simulink model "s9_10"  (Simulink 6.6)
settings: Solver=ode23  SolverMode=SingleTasking  StartTime=0.0  StopTime=t_d  MaxStep=Tc  RelTol=1e-8  AbsTol=1e-8
values from neighbouring files (symbols this model uses):
  Cp = [0 0;0 1/4e3]    [i9_10.m]
  F_v = K_r*diag([0.01 0.01])*K_r    [i9_10.m]
  g = 9.81    [i9_10.m]
  G_f = inv (S_f'*Ch*S_f)*S_f'    [i9_10.m]
  h_d = [0;- 50]    [i9_10.m]
  K_Dl = 16    [i9_10.m]
  K_Inu = 100    [i9_10.m]
  K_Pl = 100    [i9_10.m]
  K_Pnu = 16    [i9_10.m]
  o_r = [1;0]    [i9_10.m]
  pi_l = pi_m    [i9_10.m]
  pS_f = inv(S_f'*Ch*S_f)*S_f'*Ch    [i9_10.m]
  pS_v = inv(S_v'*Kh*S_v)*S_v'*Kh    [i9_10.m]
  q_i = inv_k2u(a,p_0)    [i9_10.m]
  R_c = [cos(pi/4)  -sin(pi/4) ... (first row only)    [i9_10.m]
  S_f = [0;1]    [i9_10.m]
  S_v = [1;0]    [i9_10.m]
  Tc = 0.001    [i9_10.m]
  Ts = Tc    (= 0.001)    [i9_10.m]
undefined symbols (not defined in the file or in its folder): a, DiscIntNeverNeededParam, iner, iner_l, pi_m
settings Model: Creator=luigivillani  LastModifiedBy=luigivillani  ExtModeAutoUpdateStatusClock=off
settings DataIOCC: LimitDataPoints=off  SaveOutput=off  SaveTime=off
settings OptimizationCC: BlockReduction=off  BooleanDataType=off
settings DebuggingCC: SignalResolutionControl=TryResolveAllWithWarning  SolverPrmCheckMsg=none  MultiTaskDSMMsg=warning  MultiTaskCondExecSysMsg=none  StrictBusMsg=None
settings HardwareCC: TargetUnknown=on
settings RTWCC: IncludeERTFirstTime=on

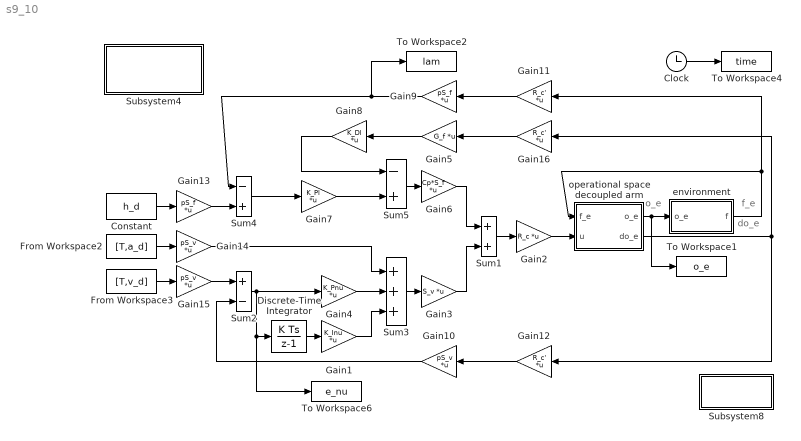
== system s9_10 ==
  note: do_e
  note: f_e
  note: o_e
  Clock : Clock
      settings: Decimation=10
  Constant : Constant  Value=h_d
  Discrete-Time Integrator : DiscreteIntegrator  SampleTime=Tc  ICPrevOutput=DiscIntNeverNeededParam  ICPrevScaledInput=DiscIntNeverNeededParam
  From Workspace2 : FromWorkspace  VariableName=[T,a_d]  SampleTime=Tc
  From Workspace3 : FromWorkspace  VariableName=[T,v_d]  SampleTime=Tc
  Gain1 : Gain  Gain=K_Inu  Multiplication=Matrix(K*u)  SampleTime=Tc
      mask Display: disp('K_Inu')
  Gain10 : Gain  Orientation=left  Gain=pS_v  Multiplication=Matrix(K*u)  SampleTime=Tc
      mask Display: disp('pS_v')
  Gain11 : Gain  Orientation=left  Gain=R_c'  Multiplication=Matrix(K*u)  SampleTime=Tc
      mask Display: disp('trR_c')
  Gain12 : Gain  Orientation=left  Gain=R_c'  Multiplication=Matrix(K*u)  SampleTime=Tc
      mask Display: disp('trR_c')
  Gain13 : Gain  Gain=pS_f  Multiplication=Matrix(K*u)  SampleTime=Tc
      mask Display: disp('pS_f')
  Gain14 : Gain  Gain=pS_v  Multiplication=Matrix(K*u)  SampleTime=Tc
      mask Display: disp('pS_v')
  Gain15 : Gain  Gain=pS_v  Multiplication=Matrix(K*u)  SampleTime=Tc
      mask Display: disp('pS_v')
  Gain16 : Gain  Orientation=left  Gain=R_c'  Multiplication=Matrix(K*u)  SampleTime=Tc
      mask Display: disp('trR_c')
  Gain2 : Gain  Gain=R_c  Multiplication=Matrix(K*u)  SampleTime=Tc
      mask Display: disp('R_c')
  Gain3 : Gain  Gain=S_v  Multiplication=Matrix(K*u)  SampleTime=Tc
      mask Display: disp('S_v')
  Gain4 : Gain  Gain=K_Pnu  Multiplication=Matrix(K*u)  SampleTime=Tc
      mask Display: disp('K_Pnu')
  Gain5 : Gain  Orientation=left  Gain=G_f  Multiplication=Matrix(K*u)  SampleTime=Tc
      mask Display: disp('G_f')
  Gain6 : Gain  Gain=Cp*S_f  Multiplication=Matrix(K*u)  SampleTime=Tc
      mask Display: disp('C''S_f')
  Gain7 : Gain  Gain=K_Pl  Multiplication=Matrix(K*u)  SampleTime=Tc
      mask Display: disp('K_Pl')
  Gain8 : Gain  Orientation=left  Gain=K_Dl  Multiplication=Matrix(K*u)  SampleTime=Tc
      mask Display: disp('K_Dl')
  Gain9 : Gain  Orientation=left  Gain=pS_f  Multiplication=Matrix(K*u)  SampleTime=Tc
      mask Display: disp('pS_f')
  Subsystem4 : Subsystem
      settings: OpenFcn=clear all;i9_10;
      mask Display: disp('variables\ninitialization')
  Subsystem8 : Subsystem  Orientation=left
      settings: OpenFcn=p9_10;
      mask Display: disp('plot')
  Sum1 : Sum  SaturateOnIntegerOverflow=on  InputSameDT=on
  Sum2 : Sum  Inputs=+-  SaturateOnIntegerOverflow=on  InputSameDT=on
  Sum3 : Sum  Inputs=+++  SaturateOnIntegerOverflow=on  InputSameDT=on
  Sum4 : Sum  Inputs=-+  SaturateOnIntegerOverflow=on  InputSameDT=on
  Sum5 : Sum  Inputs=-+  SaturateOnIntegerOverflow=on  InputSameDT=on
  To Workspace1 : ToWorkspace  VariableName=o_e  SampleTime=Ts  SaveFormat=Array
      settings: MaxDataPoints=5001
  To Workspace2 : ToWorkspace  VariableName=lam  SampleTime=Ts  SaveFormat=Array
      settings: MaxDataPoints=5001
  To Workspace4 : ToWorkspace  VariableName=time  SampleTime=Ts  SaveFormat=Array
      settings: MaxDataPoints=5001
  To Workspace6 : ToWorkspace  VariableName=e_nu  SampleTime=Ts  SaveFormat=Array
      settings: MaxDataPoints=5001
  environment : Subsystem
      mask Display: disp('K''(o_e-o_r)')
  operational space decoupled arm : Subsystem
      mask Display: disp('u = ddo_e')
  wires:
  Sum2/1 -> To Workspace6/1, Discrete-Time Integrator/1, Gain4/1
  environment/1(f) -> Gain11/1, operational space decoupled arm/1(f_e)
  Clock/1 -> To Workspace4/1
  operational space decoupled arm/1(o_e) -> environment/1(o_e), To Workspace1/1
  operational space decoupled arm/2(do_e) -> Gain12/1, Gain16/1
  Gain4/1 -> Sum3/2
  Gain2/1 -> operational space decoupled arm/2(u)
  Gain1/1 -> Sum3/3
  Discrete-Time Integrator/1 -> Gain1/1
  Sum3/1 -> Gain3/1
  Gain3/1 -> Sum1/2
  Sum4/1 -> Gain7/1
  Gain7/1 -> Sum5/2
  Sum5/1 -> Gain6/1
  Gain6/1 -> Sum1/1
  Sum1/1 -> Gain2/1
  Gain9/1 -> Sum4/1, To Workspace2/1
  Gain10/1 -> Sum2/2
  Gain5/1 -> Gain8/1
  Gain8/1 -> Sum5/1
  Gain11/1 -> Gain9/1
  Gain12/1 -> Gain10/1
  Constant/1 -> Gain13/1
  Gain13/1 -> Sum4/2
  From Workspace2/1 -> Gain14/1
  Gain14/1 -> Sum3/1
  From Workspace3/1 -> Gain15/1
  Gain15/1 -> Sum2/1
  Gain16/1 -> Gain5/1

== system s9_10/Subsystem4 ==
  note: start

== system s9_10/Subsystem8 ==
  note: start

== system s9_10/environment ==
  o_e : Inport
  Matrix gain. : StateSpace  A=[]  B=[]  C=[]  D=K  mask(Matrix gain){@1=K}
      mask prompts: @1 "Gain matrix:"
      mask help: Matrix Gain.
      mask init:
      | K = @1;
      mask Help: Multiplies input vector by entered matrix to produce output vector (y=Au).
      mask Display: disp('K')
  Sum1 : Sum  Inputs=+-  SaturateOnIntegerOverflow=on  InputSameDT=on
  xo : Constant  Value=o_r
  f : Outport  InitialOutput=0
  wires:
  xo/1 -> Sum1/2
  Sum1/1 -> Matrix gain./1
  Matrix gain./1 -> f/1
  o_e/1 -> Sum1/1

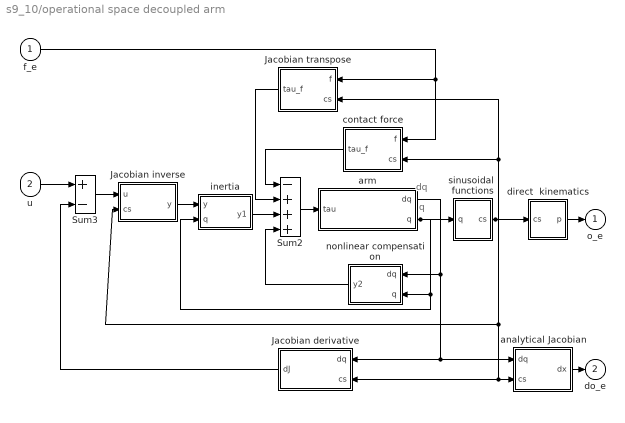
== system s9_10/operational space decoupled arm ==
  note: q
  note: dq
  f_e : Inport
  u : Inport  Port=2
  Jacobian derivative : Subsystem  Orientation=left
      mask Display: disp('dJ_a(q,dq)')
  Jacobian inverse : Subsystem
      mask Display: disp('inv(J_a(q))')
  Jacobian transpose : Subsystem  Orientation=left
      mask Display: disp('tr(J_a(q))')
  Sum2 : Sum  Inputs=-+++  SaturateOnIntegerOverflow=on  InputSameDT=on
  Sum3 : Sum  Inputs=+-  SaturateOnIntegerOverflow=on  InputSameDT=on
  analytical Jacobian : Subsystem
      mask Display: disp('J_a(q)')
  arm : Subsystem
      mask Display: disp('inv(B(q))(tau-tau'')')
  contact force : Subsystem  Orientation=left
      mask Display: disp('tr(J_a(q))f')
  direct  kinematics : Subsystem
      mask Display: disp('k(q)')
  inertia : Subsystem
      mask Display: disp('B(q)')
  nonlinear compensation : Subsystem  Orientation=left
      mask Display: disp('n(q,dq)')
  sinusoidal  functions : Subsystem
      mask Display: disp('cs(q)')
  o_e : Outport  InitialOutput=0
  do_e : Outport  Port=2  InitialOutput=0
  wires:
  Jacobian inverse/1(y) -> inertia/1(y)
  Sum2/1 -> arm/1(tau)
  arm/1(dq) -> analytical Jacobian/1(dq), Jacobian derivative/1(dq), nonlinear compensation/1(dq)
  direct  kinematics/1(p) -> o_e/1
  analytical Jacobian/1(dx) -> do_e/1
  Sum3/1 -> Jacobian inverse/1(u)
  arm/2("q ") -> sinusoidal  functions/1(q), nonlinear compensation/2(q), inertia/2(q)
  contact force/1(tau_f) -> Sum2/1
  sinusoidal  functions/1(cs) -> direct  kinematics/1(cs), contact force/2(cs), Jacobian transpose/2(cs), analytical Jacobian/2(cs), Jacobian derivative/2(cs), Jacobian inverse/2(cs)
  u/1 -> Sum3/1
  Jacobian derivative/1(dJ) -> Sum3/2
  nonlinear compensation/1(y2) -> Sum2/4
  inertia/1(y1) -> Sum2/3
  Jacobian transpose/1(tau_f) -> Sum2/2
  f_e/1 -> Jacobian transpose/1(f), contact force/1(f)

== system s9_10/operational space decoupled arm/Jacobian derivative ==
  dq : Inport
  cs : Inport  Port=2
  MATLAB Fcn : MATLABFcn  MATLABFcn=dJ_a  OutputDimensions=2  SampleTime=Tc
      mask Display: disp('dJ_a(q,dq)dq')
  Mux : Mux  Inputs=[2,4]
  dJ : Outport  InitialOutput=0
  wires:
  dq/1 -> Mux/1
  cs/1 -> Mux/2
  Mux/1 -> MATLAB Fcn/1
  MATLAB Fcn/1 -> dJ/1

== system s9_10/operational space decoupled arm/Jacobian inverse ==
  u : Inport
  cs : Inport  Port=2
  MATLAB Fcn : MATLABFcn  MATLABFcn=invJ_a  OutputDimensions=2  SampleTime=Tc
      mask Display: disp('inv(J_a(q))')
  Mux : Mux  Inputs=[2,4]
  y : Outport  InitialOutput=0
  wires:
  MATLAB Fcn/1 -> y/1
  Mux/1 -> MATLAB Fcn/1
  cs/1 -> Mux/2
  u/1 -> Mux/1

== system s9_10/operational space decoupled arm/Jacobian transpose ==
  f : Inport
  cs : Inport  Port=2
  MATLAB Fcn : MATLABFcn  MATLABFcn=trJ_a  OutputDimensions=2  SampleTime=Tc
      mask Display: disp('J''_a(q)f')
  Mux : Mux  Inputs=[2,4]
  tau_f : Outport  InitialOutput=0
  wires:
  MATLAB Fcn/1 -> tau_f/1
  Mux/1 -> MATLAB Fcn/1
  f/1 -> Mux/1
  cs/1 -> Mux/2

== system s9_10/operational space decoupled arm/analytical Jacobian ==
  dq : Inport
  cs : Inport  Port=2
  MATLAB Fcn : MATLABFcn  MATLABFcn=J_adq  OutputDimensions=2
      mask Display: disp('J_a(q)dq')
  Mux : Mux  Inputs=[2,4]
  dx : Outport  InitialOutput=0
  wires:
  dq/1 -> Mux/1
  Mux/1 -> MATLAB Fcn/1
  MATLAB Fcn/1 -> dx/1
  cs/1 -> Mux/2

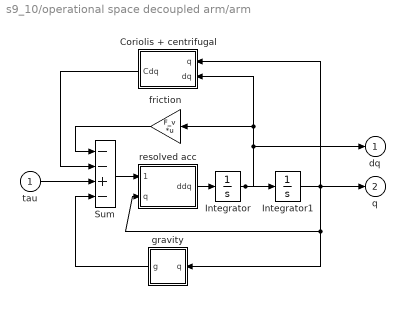
== system s9_10/operational space decoupled arm/arm ==
  tau : Inport
  Coriolis + centrifugal : Subsystem  Orientation=left
      mask Display: disp('C(q,dq)dq')
  Integrator : Integrator  InitialCondition=[0 0]  ZeroCross=off
  Integrator1 : Integrator  InitialCondition=q_i  ZeroCross=off
  Sum : Sum  Inputs=--+-  SaturateOnIntegerOverflow=on  InputSameDT=on
  friction : Gain  Orientation=left  Gain=F_v  Multiplication=Matrix(K*u)  SaturateOnIntegerOverflow=on
      mask Display: disp('F_v')
  gravity : Subsystem  Orientation=left
      mask Display: disp('g(q)')
  resolved acc : Subsystem
      mask Display: disp('inv(B(q))')
  dq : Outport  InitialOutput=0
  "q " : Outport  Port=2  InitialOutput=0
  wires:
  Coriolis + centrifugal/1(Cdq) -> Sum/2
  tau/1 -> Sum/3
  Integrator1/1 -> Coriolis + centrifugal/1(q), resolved acc/2(q), gravity/1(q), "q "/1
  resolved acc/1(ddq) -> Integrator/1
  Integrator/1 -> Integrator1/1, dq/1, Coriolis + centrifugal/2(dq), friction/1
  Sum/1 -> resolved acc/1(tau-tau')
  friction/1 -> Sum/1
  gravity/1(g) -> Sum/4

== system s9_10/operational space decoupled arm/contact force ==
  f : Inport
  cs : Inport  Port=2
  MATLAB Fcn : MATLABFcn  MATLABFcn=trJ_a  OutputDimensions=2
      mask Display: disp('J''_a(q)f')
  Mux : Mux  Inputs=[2,4]
  tau_f : Outport  InitialOutput=0
  wires:
  f/1 -> Mux/1
  cs/1 -> Mux/2
  Mux/1 -> MATLAB Fcn/1
  MATLAB Fcn/1 -> tau_f/1

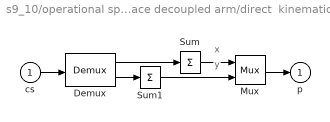
== system s9_10/operational space decoupled arm/direct  kinematics ==
  note: x
  note: y
  cs : Inport
  Demux : Demux  Outputs=[2,2]
  Mux : Mux  Inputs=2
  Sum : Sum  Inputs=+  SaturateOnIntegerOverflow=on  InputSameDT=on
  Sum1 : Sum  Inputs=+  SaturateOnIntegerOverflow=on  InputSameDT=on
  p : Outport  InitialOutput=0
  wires:
  Sum1/1 -> Mux/2
  Sum/1 -> Mux/1
  Demux/2 -> Sum1/1
  Demux/1 -> Sum/1
  cs/1 -> Demux/1
  Mux/1 -> p/1

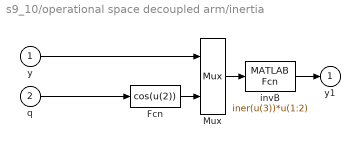
== system s9_10/operational space decoupled arm/inertia ==
  y : Inport
  q : Inport  Port=2
  Fcn : Fcn  Expr=cos(u(2))  SampleTime=Tc
  Mux : Mux  Inputs=[2,1]
  "invB " : MATLABFcn  MATLABFcn=iner(u(3))*u(1:2)  OutputDimensions=2  SampleTime=Tc
      mask Display: disp('B(q)y')
  y1 : Outport  InitialOutput=0
  wires:
  Fcn/1 -> Mux/2
  "invB "/1 -> y1/1
  Mux/1 -> "invB "/1
  q/1 -> Fcn/1
  y/1 -> Mux/1

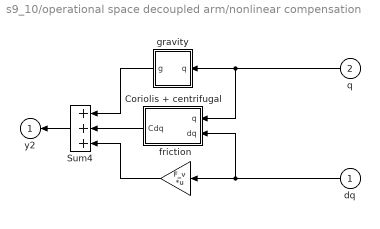
== system s9_10/operational space decoupled arm/nonlinear compensation ==
  dq : Inport  Orientation=left
  q : Inport  Orientation=left  Port=2
  Coriolis + centrifugal : Subsystem  Orientation=left
      mask Display: disp('C(q,dq)dq')
  Sum4 : Sum  Orientation=left  Inputs=+++  SaturateOnIntegerOverflow=on  InputSameDT=on
  friction : Gain  Orientation=left  Gain=F_v  Multiplication=Matrix(K*u)  SampleTime=Tc  SaturateOnIntegerOverflow=on
      mask Display: disp('F_v')
  gravity : Subsystem  Orientation=left
      mask Display: disp('g(q)')
  y2 : Outport  Orientation=left  InitialOutput=0
  wires:
  gravity/1(g) -> Sum4/1
  Sum4/1 -> y2/1
  friction/1 -> Sum4/3
  q/1 -> gravity/1(q), Coriolis + centrifugal/1(q)
  dq/1 -> Coriolis + centrifugal/2(dq), friction/1
  Coriolis + centrifugal/1(Cdq) -> Sum4/2

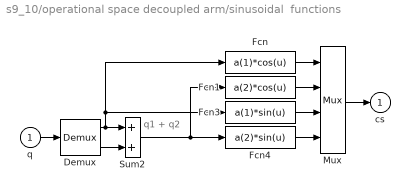
== system s9_10/operational space decoupled arm/sinusoidal  functions ==
  note: q1 + q2
  q : Inport
  Demux : Demux  Outputs=2
  Fcn : Fcn  Expr=a(1)*cos(u)
  Fcn1 : Fcn  Expr=a(2)*cos(u)
  Fcn3 : Fcn  Expr=a(1)*sin(u)
  Fcn4 : Fcn  Expr=a(2)*sin(u)
  Mux : Mux
  Sum2 : Sum  SaturateOnIntegerOverflow=on  InputSameDT=on
  cs : Outport  InitialOutput=0
  wires:
  q/1 -> Demux/1
  Fcn4/1 -> Mux/4
  Fcn3/1 -> Mux/3
  Fcn1/1 -> Mux/2
  Sum2/1 -> Fcn1/1, Fcn4/1
  Demux/2 -> Sum2/2
  Demux/1 -> Fcn/1, Fcn3/1, Sum2/1
  Mux/1 -> cs/1
  Fcn/1 -> Mux/1

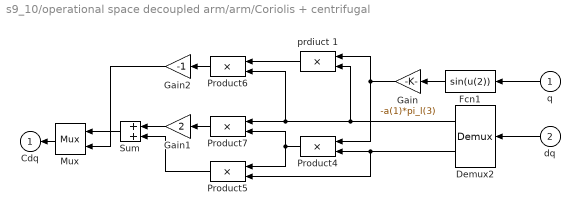
== system s9_10/operational space decoupled arm/arm/Coriolis + centrifugal ==
  q : Inport  Orientation=left
  dq : Inport  Orientation=left  Port=2
  Demux2 : Demux  Orientation=left  Outputs=2
  Fcn1 : Fcn  Orientation=left  Expr=sin(u(2))
  Gain : Gain  Orientation=left  Gain=-a(1)*pi_l(3)  SaturateOnIntegerOverflow=on
      mask Display: disp('k_3')
  Gain1 : Gain  Orientation=left  Gain=2  SaturateOnIntegerOverflow=on
  Gain2 : Gain  Orientation=left  Gain=-1  SaturateOnIntegerOverflow=on
  Mux : Mux  Orientation=left  Inputs=2
  Product{4..7} (4 alike) : Product  Orientation=left  SaturateOnIntegerOverflow=on  RndMeth=Zero  InputSameDT=on
  Sum : Sum  Orientation=left  SaturateOnIntegerOverflow=on  InputSameDT=on
  prdiuct 1 : Product  Orientation=left  SaturateOnIntegerOverflow=on  RndMeth=Zero  InputSameDT=on
  Cdq : Outport  Orientation=left  InitialOutput=0
  wires:
  dq/1 -> Demux2/1
  Gain2/1 -> Mux/2
  Product6/1 -> Gain2/1
  Mux/1 -> Cdq/1
  Sum/1 -> Mux/1
  Product5/1 -> Sum/2
  Gain1/1 -> Sum/1
  Product7/1 -> Gain1/1
  Demux2/1 -> prdiuct 1/2, Product6/2, Product7/1
  Demux2/2 -> Product4/2, Product5/2
  prdiuct 1/1 -> Product6/1
  Gain/1 -> prdiuct 1/1, Product4/1
  Fcn1/1 -> Gain/1
  q/1 -> Fcn1/1
  Product4/1 -> Product5/1, Product7/2

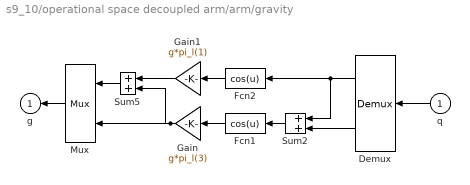
== system s9_10/operational space decoupled arm/arm/gravity ==
  q : Inport  Orientation=left
  Demux : Demux  Orientation=left  Outputs=2
  Fcn1 : Fcn  Orientation=left  Expr=cos(u)
  Fcn2 : Fcn  Orientation=left  Expr=cos(u)
  Gain : Gain  Orientation=left  Gain=g*pi_l(3)  SaturateOnIntegerOverflow=on
      mask Display: disp('k_2')
  Gain1 : Gain  Orientation=left  Gain=g*pi_l(1)  SaturateOnIntegerOverflow=on
      mask Display: disp('k_1')
  Mux : Mux  Orientation=left  Inputs=2
  Sum2 : Sum  Orientation=left  SaturateOnIntegerOverflow=on  InputSameDT=on
  Sum5 : Sum  Orientation=left  SaturateOnIntegerOverflow=on  InputSameDT=on
  g : Outport  Orientation=left  InitialOutput=0
  wires:
  q/1 -> Demux/1
  Demux/2 -> Sum2/2
  Sum2/1 -> Fcn1/1
  Fcn1/1 -> Gain/1
  Fcn2/1 -> Gain1/1
  Demux/1 -> Fcn2/1, Sum2/1
  Gain1/1 -> Sum5/1
  Sum5/1 -> Mux/1
  Gain/1 -> Sum5/2, Mux/2
  Mux/1 -> g/1

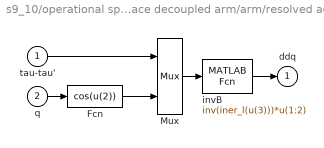
== system s9_10/operational space decoupled arm/arm/resolved acc ==
  tau-tau' : Inport
  q : Inport  Port=2
  Fcn : Fcn  Expr=cos(u(2))
  Mux : Mux  Inputs=[2,1]
  "invB " : MATLABFcn  MATLABFcn=inv(iner_l(u(3)))*u(1:2)  OutputDimensions=2
      mask Display: disp('inv(B(q))')
  ddq : Outport  InitialOutput=0
  wires:
  Fcn/1 -> Mux/2
  q/1 -> Fcn/1
  "invB "/1 -> ddq/1
  tau-tau'/1 -> Mux/1
  Mux/1 -> "invB "/1

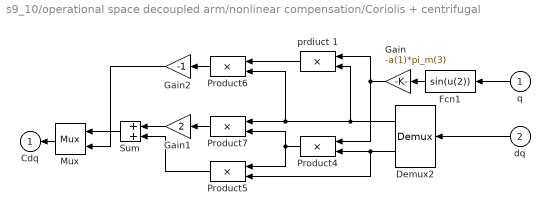
== system s9_10/operational space decoupled arm/nonlinear compensation/Coriolis + centrifugal ==
  q : Inport  Orientation=left
  dq : Inport  Orientation=left  Port=2
  Demux2 : Demux  Orientation=left  Outputs=2
  Fcn1 : Fcn  Orientation=left  Expr=sin(u(2))  SampleTime=Tc
  Gain : Gain  Orientation=left  Gain=-a(1)*pi_m(3)  SaturateOnIntegerOverflow=on
      mask Display: disp('k_3')
  Gain1 : Gain  Orientation=left  Gain=2  SaturateOnIntegerOverflow=on
  Gain2 : Gain  Orientation=left  Gain=-1  SaturateOnIntegerOverflow=on
  Mux : Mux  Orientation=left  Inputs=2
  Product{4..7} (4 alike) : Product  Orientation=left  SampleTime=Tc  SaturateOnIntegerOverflow=on  RndMeth=Zero  InputSameDT=on
  Sum : Sum  Orientation=left  SaturateOnIntegerOverflow=on  InputSameDT=on
  prdiuct 1 : Product  Orientation=left  SampleTime=Tc  SaturateOnIntegerOverflow=on  RndMeth=Zero  InputSameDT=on
  Cdq : Outport  Orientation=left  InitialOutput=0
  wires:
  Product4/1 -> Product5/1, Product7/2
  Demux2/1 -> prdiuct 1/2, Product6/2, Product7/1
  Fcn1/1 -> Gain/1
  Gain/1 -> prdiuct 1/1, Product4/1
  prdiuct 1/1 -> Product6/1
  Product7/1 -> Gain1/1
  Gain1/1 -> Sum/1
  Product5/1 -> Sum/2
  Sum/1 -> Mux/1
  Mux/1 -> Cdq/1
  Product6/1 -> Gain2/1
  Gain2/1 -> Mux/2
  q/1 -> Fcn1/1
  dq/1 -> Demux2/1
  Demux2/2 -> Product4/2, Product5/2

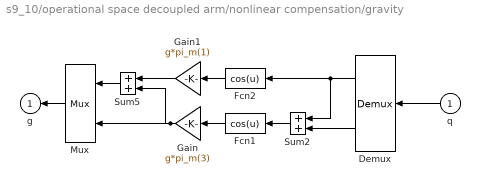
== system s9_10/operational space decoupled arm/nonlinear compensation/gravity ==
  q : Inport  Orientation=left
  Demux : Demux  Orientation=left  Outputs=2
  Fcn1 : Fcn  Orientation=left  Expr=cos(u)  SampleTime=Tc
  Fcn2 : Fcn  Orientation=left  Expr=cos(u)  SampleTime=Tc
  Gain : Gain  Orientation=left  Gain=g*pi_m(3)  SaturateOnIntegerOverflow=on
      mask Display: disp('k_2')
  Gain1 : Gain  Orientation=left  Gain=g*pi_m(1)  SaturateOnIntegerOverflow=on
      mask Display: disp('k_1')
  Mux : Mux  Orientation=left  Inputs=2
  Sum2 : Sum  Orientation=left  SampleTime=Tc  SaturateOnIntegerOverflow=on  InputSameDT=on
  Sum5 : Sum  Orientation=left  SaturateOnIntegerOverflow=on  InputSameDT=on
  g : Outport  Orientation=left  InitialOutput=0
  wires:
  q/1 -> Demux/1
  Demux/2 -> Sum2/2
  Sum2/1 -> Fcn1/1
  Fcn1/1 -> Gain/1
  Fcn2/1 -> Gain1/1
  Demux/1 -> Fcn2/1, Sum2/1
  Gain1/1 -> Sum5/1
  Sum5/1 -> Mux/1
  Gain/1 -> Mux/2, Sum5/2
  Mux/1 -> g/1
